simulink model "aerobalancin_modelo"  (R2025b)
settings: Solver=FixedStepAuto  StartTime=0.0  StopTime=20  FixedStep=1e-3  RelTol=1e-3
values from neighbouring files (symbols this model uses):
  d1 = 130.5e-3    (= 0.1305)    [Fuerzas.m]    (also in modelo_no_lineal.m; smc_proyecto.m)
  I = 1.3636e-4    (= 0.00013636)    [Fuerzas.m]    (also in modelo_no_lineal.m; smc_proyecto.m)
  k = (Wcp*d2-d1*Wm-e*Wb)    (= -0.00869250366)    [Fuerzas.m]    (also in modelo_no_lineal.m; smc_proyecto.m)
  mu = 2e-04    (= 0.0002)    [Fuerzas.m]    (also in modelo_no_lineal.m = 0.0007406734; smc_proyecto.m = 0.0004406734)
libraries: simulink_extras x1
settings Model: Creator=Gabriel Bojaca  LastModifiedBy=Gabriel Bojaca

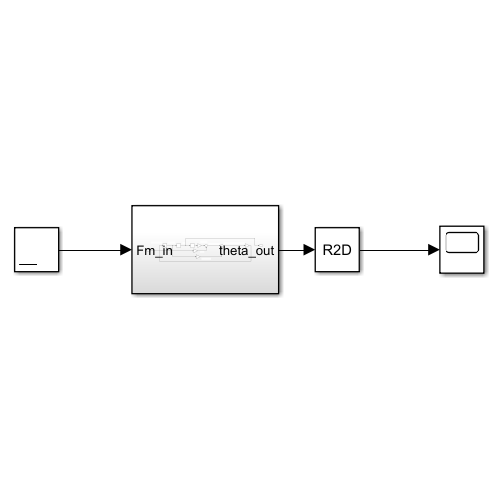
[thumbnail: Simulink's stored preview of the top-level diagram]
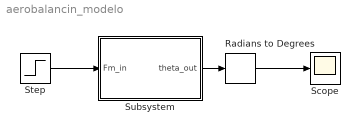
== system aerobalancin_modelo ==
  Radians to Degrees : simulink_extras/Transformations/Radians to Degrees
  Scope : Scope
      settings: ActiveDisplayYMinimum=-7.9335291049112415  ActiveDisplayYMaximum=71.401761944201183
  Step : Step  After=50e-3  SampleTime=0
  Subsystem : Subsystem
  wires:
  Subsystem/1(theta_out) -> Radians to Degrees/1
  Step/1 -> Subsystem/1(Fm_in)
  Radians to Degrees/1 -> Scope/1

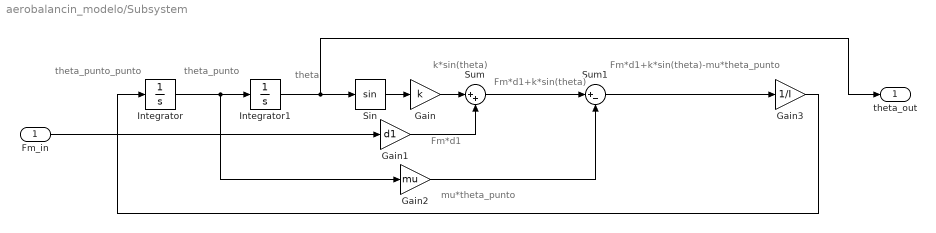
== system aerobalancin_modelo/Subsystem ==
  note: Fm*d1
  note: k*sin(theta)
  note: theta_punto_punto
  note: theta_punto
  note: theta
  note: Fm*d1+k*sin(theta)
  note: mu*theta_punto
  note: Fm*d1+k*sin(theta)-mu*theta_punto
  Fm_in : Inport
  Gain : Gain  Gain=k
  Gain1 : Gain  Gain=d1
  Gain2 : Gain  Gain=mu
  Gain3 : Gain  Gain=1/I
  Integrator : Integrator
  Integrator1 : Integrator
  Sin : Trigonometry
  Sum : Sum  Inputs=|++
  Sum1 : Sum  Inputs=|+-
  theta_out : Outport
  wires:
  Sum1/1 -> Gain3/1
  Gain3/1 -> Integrator/1
  Sin/1 -> Gain/1
  Integrator/1 -> Gain2/1, Integrator1/1
  Integrator1/1 -> theta_out/1, Sin/1
  Gain/1 -> Sum/1
  Sum/1 -> Sum1/1
  Gain2/1 -> Sum1/2
  Gain1/1 -> Sum/2
  Fm_in/1 -> Gain1/1
